simulink model "get_jac_test"  (R2022a)
settings: Solver=VariableStepAuto  StartTime=0.0  StopTime=1  RelTol=1e-3
values from neighbouring files (symbols this model uses):
  sc = SpaceRobot    [model_test.m]    (also in test.m = SpaceRobot('SC_2DoF.urdf'))
settings Model: Creator=charl  LastModifiedBy=charl

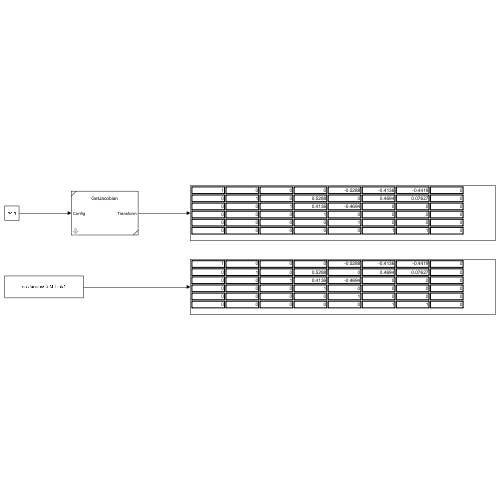
[thumbnail: Simulink's stored preview of the top-level diagram]
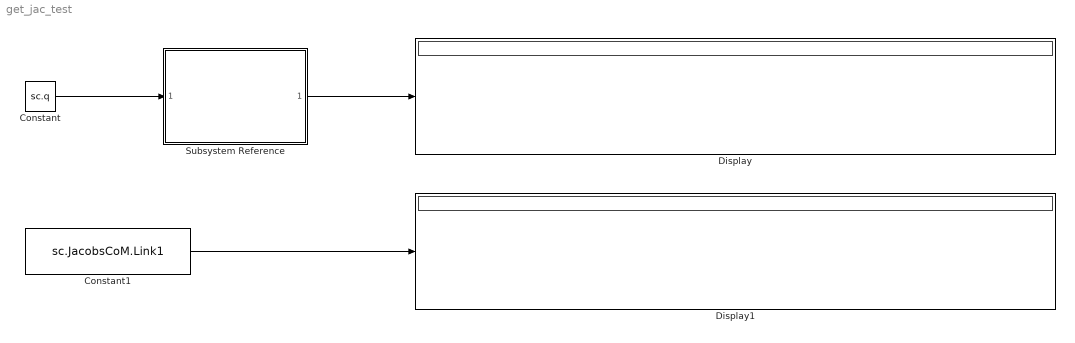
== system get_jac_test ==
  Constant : Constant  Value=sc.q
  Constant1 : Constant  Value=sc.JacobsCoM.Link1
  Display : Display
  Display1 : Display
  Subsystem Reference : Subsystem  ReferencedSubsystem=GetJacobian  spaceRobot=sc  sourceLink=Link1  SimulateUsing=Interpreted execution
  wires:
  Subsystem Reference/1 -> Display/1
  Constant/1 -> Subsystem Reference/1
  Constant1/1 -> Display1/1
